simulink model "gm_sampleModel2055_3_sub"  (R2023a)
settings: Solver=VariableStepAuto  StartTime=0.0  StopTime=10.0  RelTol=1e-3
libraries: simulink x3
settings Model: Creator=user1  LastModifiedBy=user1
settings OptimizationCC: BlockReduction=off  ConditionallyExecuteInputs=off
settings DebuggingCC: InheritedTsInSrcMsg=none

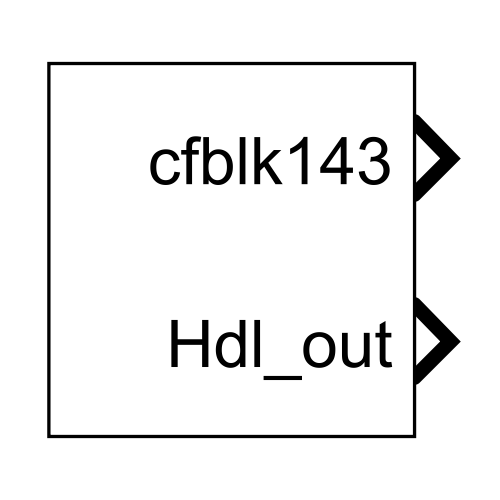
[thumbnail: Simulink's stored preview of the top-level diagram]
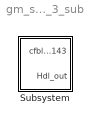
== system gm_sampleModel2055_3_sub ==
  Subsystem : Subsystem

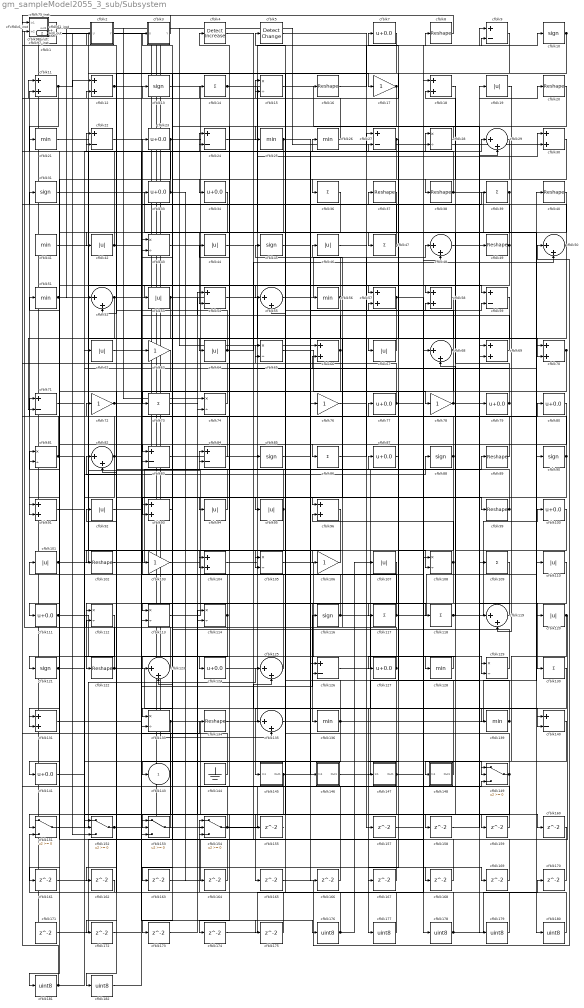
== system gm_sampleModel2055_3_sub/Subsystem ==
  cfblk1 : simulink/Logic and Bit Operations/Detect Decrease  vinit=0.0  OutDataTypeStr=uint8
      settings: LibrarySourceBlock=|
      | hdlsllib/Logic and Bit
      | Operations/Detect
      | Decrease
  cfblk{10,13,31,45,85,88,90,116,121} (9 alike) : Signum
  cfblk{7,23,33..34,77,79..80,87,100,111,124,127,141} (13 alike) : Bias  Bias=0.0  SaturateOnIntegerOverflow=off
  cfblk{19,42,44,46,53,62,64,67,92,94..95,101,107,110,120} (15 alike) : Abs  OutDataTypeStr=uint8  SaturateOnIntegerOverflow=off
  cfblk{8,16,20,37..38,40,49,89,99,102,122,134} (12 alike) : Reshape
  cfblk{17,63,72,76,78,103,106} (7 alike) : Gain  OutDataTypeStr=uint8
  cfblk{11..12,18,30,57..58,66,69..70,91,93,96,104,131} (14 alike) : Sum  OutDataTypeStr=uint8
  cfblk{15,28,43,65,74,81,105,108,112..114,129,133} (13 alike) : Product  Inputs=*/  OutDataTypeStr=uint8  RndMeth=Zero  SaturateOnIntegerOverflow=on
  cfblk{14,36,39,47,73,86,109,117..118,130} (10 alike) : Sum  Inputs=+  OutDataTypeStr=uint8
  cfblk115_inst : Subsystem
  cfblk{29,48,50,52,55,68,82,119,123,125,135} (11 alike) : Sum  Inputs=|++  OutDataTypeStr=uint8
  cfblk{9,22,24,27,54,59,71,83..84,126,140} (11 alike) : Sum  Inputs=+-  OutDataTypeStr=uint8
  cfblk{21,25..26,41,51,56,128,136,139} (9 alike) : MinMax  OutDataTypeStr=uint8
  cfblk144 : Ground
  cfblk145 : Subsystem
  cfblk146 : Subsystem
  cfblk147 : Subsystem
  cfblk148 : Subsystem
  cfblk{149,151..154} (5 alike) : Switch  OutDataTypeStr=uint8  SaturateOnIntegerOverflow=off  InputSameDT=off
  cfblk{155,157..175} (20 alike) : Delay  SampleTime=1
  cfblk{176..182} (7 alike) : DataTypeConversion  OutDataTypeStr=uint8  SaturateOnIntegerOverflow=off  RndMeth=Floor
  cfblk2 : Subsystem  mask(Detect Fall Nonpositive){vinit=double(0), InputProcessing=Elements as channels (sample based), OutDataTypeStr=uint8}
      mask prompts: vinit "Simulink:masks:InitialCondition_MP"; InputProcessing "Simulink:masks:InputProcessing_MP"; OutDataTypeStr "Simulink:masks:OutputDataType_MP"
      mask help: Simulink:masks:DetectFallNonpositive_MD
      mask init:
      | InputProcessing = 'Elements as channels (sample based)';
      | OutDataTypeStr = 'uint8';
      | vinit = double(0);
      mask TypeOptions InputProcessing: Simulink:masks:ColumnsAsChannelsFrameBased | Simulink:masks:ElementsAsChannelsSampleBased
      mask TypeOptions OutDataTypeStr: Simulink:masks:uint8 | Simulink:masks:boolean
      mask Display: fprintf('U <= 0\n&  NOT\nU/z <= 0')
  cfblk3 : Subsystem  mask(Detect Fall Negative){vinit=double(0), InputProcessing=Elements as channels (sample based), OutDataTypeStr=uint8}
      mask prompts: vinit "Simulink:masks:InitialCondition_MP"; InputProcessing "Simulink:masks:InputProcessing_MP"; OutDataTypeStr "Simulink:masks:OutputDataType_MP"
      mask help: Simulink:masks:DetectFallNegative_MD
      mask init:
      | InputProcessing = 'Elements as channels (sample based)';
      | OutDataTypeStr = 'uint8';
      | vinit = double(0);
      mask TypeOptions InputProcessing: Simulink:masks:ColumnsAsChannelsFrameBased | Simulink:masks:ElementsAsChannelsSampleBased
      mask TypeOptions OutDataTypeStr: Simulink:masks:uint8 | Simulink:masks:boolean
      mask Display: fprintf('U < 0\n&  NOT\nU/z < 0')
  cfblk32_inst : Subsystem
  cfblk35_inst : Subsystem
  cfblk4 : simulink/Logic and Bit Operations/Detect Increase  vinit=0.0  OutDataTypeStr=uint8
      settings: LibrarySourceBlock=|
      | hdlsllib/Logic and Bit
      | Operations/Detect
      | Increase
  cfblk5 : simulink/Logic and Bit Operations/Detect Change  vinit=0  OutDataTypeStr=uint8
      settings: LibrarySourceBlock=|
      | hdlsllib/Logic and Bit
      | Operations/Detect
      | Change
  cfblk60_inst : Subsystem
  cfblk61_inst : Subsystem
  cfblk6_inst : Subsystem
  cfblk75_inst : Subsystem
  cfblk97_inst : Subsystem
  cfblk98_inst : Subsystem
  cfblk143 : Outport  OutDataTypeStr=uint8  SampleTime=1  VectorParamsAs1DForOutWhenUnconnected=off
  Hdl_out : Outport  Port=2  OutDataTypeStr=uint8  SampleTime=1
  wires:
  cfblk1/1 -> cfblk152/3, cfblk17/1, cfblk108/2
  cfblk10/1 -> cfblk13/1, cfblk133/1
  cfblk100/1 -> cfblk153/2
  cfblk101/1 -> cfblk84/1, cfblk28/1
  cfblk102/1 -> cfblk89/1
  cfblk103/1 -> cfblk87/1
  cfblk104/1 -> cfblk80/1
  cfblk105/1 -> cfblk129/2
  cfblk106/1 -> cfblk102/1
  cfblk107/1 -> cfblk136/1
  cfblk108/1 -> cfblk96/2, cfblk153/1
  cfblk109/1 -> cfblk122/1
  cfblk11/1 -> cfblk91/2, cfblk12/1
  cfblk110/1 -> cfblk130/1
  cfblk111/1 -> cfblk71/1, cfblk129/1
  cfblk112/1 -> cfblk121/1
  cfblk113/1 -> cfblk29/2
  cfblk114/1 -> cfblk81/1, cfblk133/2
  cfblk115_inst/1(out1) -> cfblk74/1
  cfblk116/1 -> cfblk82/2, cfblk140/2
  cfblk117/1 -> cfblk55/2, cfblk40/1
  cfblk118/1 -> cfblk68/2, cfblk100/1
  cfblk119/1 -> cfblk112/1
  cfblk12/1 -> cfblk52/2, cfblk168/1
  cfblk120/1 -> cfblk154/1, cfblk149/2
  cfblk121/1 -> cfblk149/1, cfblk26/1
  cfblk122/1 -> cfblk177/1, cfblk51/1
  cfblk123/1 -> cfblk22/1
  cfblk124/1 -> cfblk30/1
  cfblk125/1 -> cfblk23/1
  cfblk126/1 -> cfblk19/1
  cfblk127/1 -> cfblk61_inst/2(in2), cfblk46/1
  cfblk128/1 -> cfblk127/1
  cfblk129/1 -> cfblk3/1(U)
  cfblk13/1 -> cfblk146/1(In1)
  cfblk130/1 -> cfblk145/1(In1)
  cfblk131/1 -> cfblk108/1
  cfblk133/1 -> cfblk182/1, cfblk165/1
  cfblk134/1 -> cfblk9/2
  cfblk135/1 -> cfblk29/1
  cfblk136/1 -> cfblk90/1, cfblk45/1, cfblk173/1
  cfblk139/1 -> cfblk37/1, cfblk116/1
  cfblk14/1 -> cfblk180/1, cfblk47/1
  cfblk140/1 -> cfblk148/1(In1)
  cfblk141/1 -> cfblk62/1
  cfblk144/1 -> cfblk75_inst/1(in1)
  cfblk145/1(Out1) -> cfblk58/2, cfblk174/1
  cfblk146/1(Out1) -> cfblk49/1
  cfblk147/1(Out1) -> cfblk9/1, cfblk84/2, cfblk163/1
  cfblk148/1(Out1) -> cfblk5/1
  cfblk149/1 -> cfblk151/2, cfblk101/1
  cfblk15/1 -> cfblk109/1
  cfblk151/1 -> cfblk125/1
  cfblk152/1 -> cfblk77/1, cfblk134/1
  cfblk153/1 -> cfblk98_inst/2(in2)
  cfblk154/1 -> cfblk79/1, cfblk72/1
  cfblk155/1 -> cfblk1/1
  cfblk157/1 -> cfblk68/1
  cfblk158/1 -> cfblk119/1
  cfblk159/1 -> cfblk32_inst/1(in1)
  cfblk16/1 -> cfblk8/1
  cfblk160/1 -> cfblk154/2
  cfblk161/1 -> cfblk125/2
  cfblk162/1 -> cfblk151/3
  cfblk163/1 -> cfblk28/2
  cfblk164/1 -> cfblk81/2
  cfblk165/1 -> cfblk50/1
  cfblk166/1 -> cfblk24/1
  cfblk167/1 -> cfblk83/2
  cfblk168/1 -> cfblk43/2
  cfblk169/1 -> cfblk82/1
  cfblk17/1 -> cfblk93/2, cfblk83/1
  cfblk170/1 -> cfblk112/2
  cfblk171/1 -> cfblk114/1
  cfblk172/1 -> cfblk126/2
  cfblk173/1 -> cfblk149/3
  cfblk174/1 -> cfblk48/2
  cfblk175/1 -> cfblk154/3
  cfblk176/1 -> cfblk92/1, cfblk107/1
  cfblk177/1 -> cfblk2/1(U)
  cfblk178/1 -> cfblk152/1, cfblk170/1
  cfblk179/1 -> cfblk65/1
  cfblk18/1 -> cfblk38/1
  cfblk180/1 -> cfblk65/2
  cfblk181/1 -> cfblk97_inst/2(in2), cfblk88/1
  cfblk182/1 -> cfblk63/1
  cfblk19/1 -> cfblk119/2
  cfblk2/1(Y) -> cfblk176/1
  cfblk20/1 -> cfblk34/1
  cfblk21/1 -> cfblk58/1
  cfblk22/1 -> cfblk117/1
  cfblk23/1 -> cfblk27/2, cfblk141/1
  cfblk24/1 -> cfblk10/1
  cfblk25/1 -> cfblk59/1, cfblk123/1
  cfblk26/1 -> cfblk115_inst/1(in1)
  cfblk27/1 -> cfblk67/1, cfblk104/2
  cfblk28/1 -> cfblk25/1
  cfblk29/1 -> cfblk93/1
  cfblk3/1(Y) -> cfblk97_inst/1(in1)
  cfblk30/1 -> cfblk36/1
  cfblk31/1 -> cfblk166/1
  cfblk32_inst/1(out1) -> cfblk151/1
  cfblk33/1 -> cfblk61_inst/1(in1), cfblk164/1
  cfblk34/1 -> cfblk111/1
  cfblk35_inst/1(out1) -> cfblk66/1
  cfblk36/1 -> cfblk155/1
  cfblk37/1 -> cfblk54/2
  cfblk38/1 -> cfblk98_inst/1(in1), cfblk110/1
  cfblk39/1 -> cfblk113/1, cfblk73/1
  cfblk4/1 -> cfblk99/1
  cfblk40/1 -> cfblk128/1
  cfblk41/1 -> cfblk179/1
  cfblk42/1 -> cfblk94/1, cfblk11/2
  cfblk43/1 -> cfblk126/1
  cfblk44/1 -> cfblk139/1
  cfblk45/1 -> cfblk70/2
  cfblk46/1 -> cfblk78/1
  cfblk47/1 -> cfblk6_inst/2(in2), cfblk24/2
  cfblk48/1 -> cfblk120/1
  cfblk49/1 -> cfblk91/1, cfblk7/1
  cfblk5/1 -> cfblk157/1
  cfblk50/1 -> cfblk105/2, cfblk14/1
  cfblk51/1 -> cfblk20/1, cfblk114/2
  cfblk52/1 -> cfblk71/2, cfblk57/1
  cfblk53/1 -> cfblk161/1, cfblk160/1
  cfblk54/1 -> cfblk76/1
  cfblk55/1 -> cfblk18/1
  cfblk56/1 -> cfblk55/1, cfblk15/1, cfblk103/1
  cfblk57/1 -> cfblk153/3, cfblk159/1
  cfblk58/1 -> cfblk131/2
  cfblk59/1 -> cfblk96/1
  cfblk6_inst/1(out1) -> cfblk52/1, cfblk115_inst/2(in2)
  cfblk60_inst/1(out1) -> cfblk171/1
  cfblk61_inst/1(out1) -> cfblk85/1, cfblk135/2
  cfblk62/1 -> cfblk74/2
  cfblk63/1 -> cfblk181/1
  cfblk64/1 -> cfblk60_inst/2(in2), cfblk50/2
  cfblk65/1 -> cfblk178/1
  cfblk66/1 -> cfblk53/1, cfblk162/1
  cfblk67/1 -> cfblk64/1
  cfblk68/1 -> cfblk11/1, cfblk15/2, cfblk86/1
  cfblk69/1 -> cfblk54/1
  cfblk7/1 -> cfblk42/1
  cfblk70/1 -> cfblk135/1, cfblk147/1(In1)
  cfblk71/1 -> cfblk70/1
  cfblk72/1 -> cfblk95/1, cfblk39/1
  cfblk73/1 -> cfblk106/1
  cfblk74/1 -> cfblk21/1
  cfblk75_inst/1(out1) -> cfblk60_inst/1(in1), cfblk41/1, cfblk56/1
  cfblk76/1 -> cfblk140/1
  cfblk77/1 -> cfblk35_inst/2(in2), cfblk169/1
  cfblk78/1 -> cfblk69/2, cfblk44/1
  cfblk79/1 -> cfblk66/2, cfblk18/2
  cfblk8/1 -> cfblk35_inst/1(in1)
  cfblk80/1 -> cfblk131/1
  cfblk81/1 -> cfblk32_inst/2(in2), cfblk104/1, cfblk158/1
  cfblk82/1 -> cfblk75_inst/2(in2), cfblk152/2, cfblk175/1
  cfblk83/1 -> cfblk118/1
  cfblk84/1 -> cfblk33/1
  cfblk85/1 -> cfblk59/2
  cfblk86/1 -> cfblk48/1
  cfblk87/1 -> cfblk57/2
  cfblk88/1 -> cfblk31/1, cfblk167/1
  cfblk89/1 -> cfblk22/2
  cfblk9/1 -> cfblk105/1
  cfblk90/1 -> cfblk69/1, cfblk172/1
  cfblk91/1 -> cfblk124/1
  cfblk92/1 -> cfblk27/1
  cfblk93/1 -> cfblk143/1
  cfblk94/1 -> cfblk6_inst/1(in1)
  cfblk95/1 -> cfblk123/2, cfblk4/1
  cfblk96/1 -> cfblk113/2
  cfblk97_inst/1(out1) -> cfblk16/1
  cfblk98_inst/1(out1) -> cfblk30/2, Hdl_out/1
  cfblk99/1 -> cfblk12/2, cfblk43/1

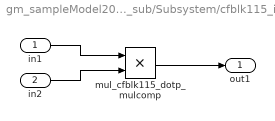
== system gm_sampleModel2055_3_sub/Subsystem/cfblk115_inst ==
  in1 : Inport  OutDataTypeStr=uint8  SampleTime=1
  in2 : Inport  Port=2  OutDataTypeStr=uint8  SampleTime=1
  mul_cfblk115_dotp_mulcomp : Product  Inputs=**  OutDataTypeStr=uint8  SampleTime=1
  out1 : Outport  OutDataTypeStr=uint8  SampleTime=1
  wires:
  in1/1 -> mul_cfblk115_dotp_mulcomp/1
  in2/1 -> mul_cfblk115_dotp_mulcomp/2
  mul_cfblk115_dotp_mulcomp/1 -> out1/1

== system gm_sampleModel2055_3_sub/Subsystem/cfblk145 ==
  In1 : Inport  OutDataTypeStr=uint8  PortDimensions=1  SampleTime=1
  Out1 : Outport  SampleTime=1
  wires:
  In1/1 -> Out1/1

== system gm_sampleModel2055_3_sub/Subsystem/cfblk146 ==
  In1 : Inport  OutDataTypeStr=uint8  PortDimensions=1  SampleTime=1
  Out1 : Outport  SampleTime=1
  wires:
  In1/1 -> Out1/1

== system gm_sampleModel2055_3_sub/Subsystem/cfblk147 ==
  In1 : Inport  OutDataTypeStr=uint8  PortDimensions=1  SampleTime=1
  Out1 : Outport  SampleTime=1
  wires:
  In1/1 -> Out1/1

== system gm_sampleModel2055_3_sub/Subsystem/cfblk148 ==
  In1 : Inport  OutDataTypeStr=uint8  PortDimensions=1  SampleTime=1
  Out1 : Outport  SampleTime=1
  wires:
  In1/1 -> Out1/1

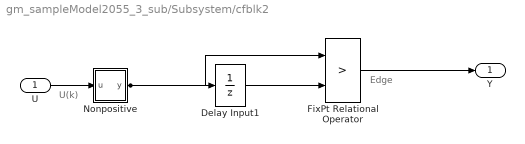
== system gm_sampleModel2055_3_sub/Subsystem/cfblk2 ==
  note: U(k)
  note: Edge
  U : Inport  OutDataTypeStr=uint8  SampleTime=1
  Delay Input1 : UnitDelay  Description=Store in Global RAM  DisableCoverage=on  InitialCondition=vinit  SampleTime=-1  HasFrameUpgradeWarning=on
  FixPt Relational Operator : RelationalOperator  Operator=>  OutDataTypeStr=fixdt(0, 8)  ZeroCross=off  InputSameDT=off
  Nonpositive : Subsystem  mask(Compare To Zero){relop=<=, OutDataTypeStr=boolean, ZeroCross=off}
      mask prompts: relop "Simulink:masks:Operator_MP"; OutDataTypeStr "Simulink:masks:OutputDataType_MP"; ZeroCross "Simulink:masks:EnableZerocrossingDetection_MP"
      mask help: Simulink:masks:CompareToZero_MD
      mask init:
      | OutDataTypeStr = 'boolean';
      | ZeroCross = 'off';
      | blkName = 'sampleModel2055_3_sub/Subsystem/cfblk2/Nonpositive';
      | relop = '<=';
      | setValue = 'boolean';
      mask TypeOptions relop: == | ~= | < | <= | >= | >
      mask TypeOptions OutDataTypeStr: Simulink:masks:uint8 | Simulink:masks:boolean
      mask Callback ZeroCross: sl('zeroCrossEnable', gcbh);
      mask Display: disp([relop,' 0'])
  Y : Outport  SampleTime=1
  wires:
  U/1 -> Nonpositive/1(u)
  Delay Input1/1 -> FixPt Relational Operator/2
  FixPt Relational Operator/1 -> Y/1
  Nonpositive/1(y) -> FixPt Relational Operator/1, Delay Input1/1

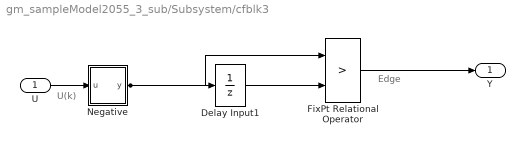
== system gm_sampleModel2055_3_sub/Subsystem/cfblk3 ==
  note: U(k)
  note: Edge
  U : Inport  OutDataTypeStr=uint8  SampleTime=1
  Delay Input1 : UnitDelay  Description=Store in Global RAM  DisableCoverage=on  InitialCondition=vinit  SampleTime=-1  HasFrameUpgradeWarning=on
  FixPt Relational Operator : RelationalOperator  Operator=>  OutDataTypeStr=fixdt(0, 8)  ZeroCross=off  InputSameDT=off
  Negative : Subsystem  mask(Compare To Zero){relop=<, OutDataTypeStr=boolean, ZeroCross=off}
      mask prompts: relop "Simulink:masks:Operator_MP"; OutDataTypeStr "Simulink:masks:OutputDataType_MP"; ZeroCross "Simulink:masks:EnableZerocrossingDetection_MP"
      mask help: Simulink:masks:CompareToZero_MD
      mask init:
      | OutDataTypeStr = 'boolean';
      | ZeroCross = 'off';
      | blkName = 'sampleModel2055_3_sub/Subsystem/cfblk3/Negative';
      | relop = '<';
      | setValue = 'boolean';
      mask TypeOptions relop: == | ~= | < | <= | >= | >
      mask TypeOptions OutDataTypeStr: Simulink:masks:uint8 | Simulink:masks:boolean
      mask Callback ZeroCross: sl('zeroCrossEnable', gcbh);
      mask Display: disp([relop,' 0'])
  Y : Outport  SampleTime=1
  wires:
  U/1 -> Negative/1(u)
  Delay Input1/1 -> FixPt Relational Operator/2
  FixPt Relational Operator/1 -> Y/1
  Negative/1(y) -> FixPt Relational Operator/1, Delay Input1/1

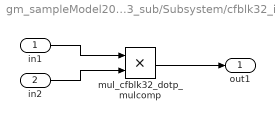
== system gm_sampleModel2055_3_sub/Subsystem/cfblk32_inst ==
  in1 : Inport  OutDataTypeStr=uint8  SampleTime=1
  in2 : Inport  Port=2  OutDataTypeStr=uint8  SampleTime=1
  mul_cfblk32_dotp_mulcomp : Product  Inputs=**  OutDataTypeStr=uint8  SampleTime=1
  out1 : Outport  OutDataTypeStr=uint8  SampleTime=1
  wires:
  in1/1 -> mul_cfblk32_dotp_mulcomp/1
  in2/1 -> mul_cfblk32_dotp_mulcomp/2
  mul_cfblk32_dotp_mulcomp/1 -> out1/1

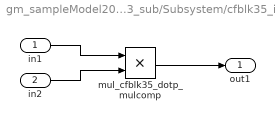
== system gm_sampleModel2055_3_sub/Subsystem/cfblk35_inst ==
  in1 : Inport  OutDataTypeStr=uint8  SampleTime=1
  in2 : Inport  Port=2  OutDataTypeStr=uint8  SampleTime=1
  mul_cfblk35_dotp_mulcomp : Product  Inputs=**  OutDataTypeStr=uint8  SampleTime=1
  out1 : Outport  OutDataTypeStr=uint8  SampleTime=1
  wires:
  in1/1 -> mul_cfblk35_dotp_mulcomp/1
  in2/1 -> mul_cfblk35_dotp_mulcomp/2
  mul_cfblk35_dotp_mulcomp/1 -> out1/1

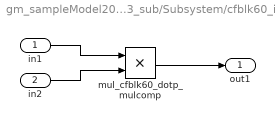
== system gm_sampleModel2055_3_sub/Subsystem/cfblk60_inst ==
  in1 : Inport  OutDataTypeStr=uint8  SampleTime=1
  in2 : Inport  Port=2  OutDataTypeStr=uint8  SampleTime=1
  mul_cfblk60_dotp_mulcomp : Product  Inputs=**  OutDataTypeStr=uint8  SampleTime=1
  out1 : Outport  OutDataTypeStr=uint8  SampleTime=1
  wires:
  in1/1 -> mul_cfblk60_dotp_mulcomp/1
  in2/1 -> mul_cfblk60_dotp_mulcomp/2
  mul_cfblk60_dotp_mulcomp/1 -> out1/1

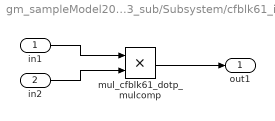
== system gm_sampleModel2055_3_sub/Subsystem/cfblk61_inst ==
  in1 : Inport  OutDataTypeStr=uint8  SampleTime=1
  in2 : Inport  Port=2  OutDataTypeStr=uint8  SampleTime=1
  mul_cfblk61_dotp_mulcomp : Product  Inputs=**  OutDataTypeStr=uint8  SampleTime=1
  out1 : Outport  OutDataTypeStr=uint8  SampleTime=1
  wires:
  in1/1 -> mul_cfblk61_dotp_mulcomp/1
  in2/1 -> mul_cfblk61_dotp_mulcomp/2
  mul_cfblk61_dotp_mulcomp/1 -> out1/1

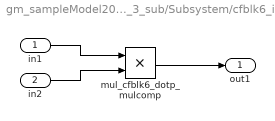
== system gm_sampleModel2055_3_sub/Subsystem/cfblk6_inst ==
  in1 : Inport  OutDataTypeStr=uint8  SampleTime=1
  in2 : Inport  Port=2  OutDataTypeStr=uint8  SampleTime=1
  mul_cfblk6_dotp_mulcomp : Product  Inputs=**  OutDataTypeStr=uint8  SampleTime=1
  out1 : Outport  OutDataTypeStr=uint8  SampleTime=1
  wires:
  in1/1 -> mul_cfblk6_dotp_mulcomp/1
  in2/1 -> mul_cfblk6_dotp_mulcomp/2
  mul_cfblk6_dotp_mulcomp/1 -> out1/1

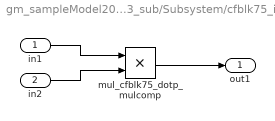
== system gm_sampleModel2055_3_sub/Subsystem/cfblk75_inst ==
  in1 : Inport  OutDataTypeStr=uint8  SampleTime=1
  in2 : Inport  Port=2  OutDataTypeStr=uint8  SampleTime=1
  mul_cfblk75_dotp_mulcomp : Product  Inputs=**  OutDataTypeStr=uint8  SampleTime=1
  out1 : Outport  OutDataTypeStr=uint8  SampleTime=1
  wires:
  in1/1 -> mul_cfblk75_dotp_mulcomp/1
  in2/1 -> mul_cfblk75_dotp_mulcomp/2
  mul_cfblk75_dotp_mulcomp/1 -> out1/1

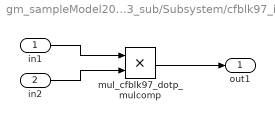
== system gm_sampleModel2055_3_sub/Subsystem/cfblk97_inst ==
  in1 : Inport  OutDataTypeStr=uint8  SampleTime=1
  in2 : Inport  Port=2  OutDataTypeStr=uint8  SampleTime=1
  mul_cfblk97_dotp_mulcomp : Product  Inputs=**  OutDataTypeStr=uint8  SampleTime=1
  out1 : Outport  OutDataTypeStr=uint8  SampleTime=1
  wires:
  in1/1 -> mul_cfblk97_dotp_mulcomp/1
  in2/1 -> mul_cfblk97_dotp_mulcomp/2
  mul_cfblk97_dotp_mulcomp/1 -> out1/1

== system gm_sampleModel2055_3_sub/Subsystem/cfblk98_inst ==
  in1 : Inport  OutDataTypeStr=uint8  SampleTime=1
  in2 : Inport  Port=2  OutDataTypeStr=uint8  SampleTime=1
  mul_cfblk98_dotp_mulcomp : Product  Inputs=**  OutDataTypeStr=uint8  SampleTime=1
  out1 : Outport  OutDataTypeStr=uint8  SampleTime=1
  wires:
  in1/1 -> mul_cfblk98_dotp_mulcomp/1
  in2/1 -> mul_cfblk98_dotp_mulcomp/2
  mul_cfblk98_dotp_mulcomp/1 -> out1/1

== system gm_sampleModel2055_3_sub/Subsystem/cfblk2/Nonpositive ==
  u : Inport  OutDataTypeStr=uint8  SampleTime=1
  Compare : RelationalOperator  Operator=<=  OutDataTypeStr=boolean  ZeroCross=off
  Constant : Constant  DisableCoverage=on  Value=0  OutDataTypeStr=Inherit: Inherit via back propagation  SampleTime=-1  PreserveConstantTs=on
  y : Outport  SampleTime=1
  wires:
  u/1 -> Compare/1
  Compare/1 -> y/1
  Constant/1 -> Compare/2

== system gm_sampleModel2055_3_sub/Subsystem/cfblk3/Negative ==
  u : Inport  OutDataTypeStr=uint8  SampleTime=1
  Compare : RelationalOperator  Operator=<  OutDataTypeStr=boolean  ZeroCross=off
  Constant : Constant  DisableCoverage=on  Value=0  OutDataTypeStr=Inherit: Inherit via back propagation  SampleTime=-1  PreserveConstantTs=on
  y : Outport  SampleTime=1
  wires:
  u/1 -> Compare/1
  Compare/1 -> y/1
  Constant/1 -> Compare/2
